simulink model "TeamA_PAsqualo"  (R2020a)
settings: Solver=VariableStepAuto  StartTime=0.0  StopTime=stop_time  FixedStep=0.05  RelTol=1e-3
InitFcn:
  | main_init
values from neighbouring files (symbols this model uses):
  a1 = rho * D^4 * alpha1    (= 0.000388302366464)    [main_init.m]
  a2 = -rho * D^3 * alpha2 * (1 - omega)    (= 0.0037030698432)    [main_init.m]
  ag = [Ax Ay Az]'    [init_modello.m]
  alpha1 = 0.0113    [main_init.m]
  alpha2 = -0.0091    [main_init.m]
  areaOfInterestCorner = [42.317744;10.915136; 0]    [init_controllo.m]    (also in missionA.m = [42.317744)
  bg = [Bx By Bz]'    [init_modello.m]
  cd_pitch = 0.7    [init_modello.m]
  cd_roll = 0.04    [init_modello.m]
  cd_x = 0.4    [init_modello.m]
  cd_y = 1    [init_modello.m]
  cd_yaw = 0.7    [init_modello.m]
  cd_z = 1    [init_modello.m]
  cg = [Cx Cy Cz]'    [init_modello.m]
  D = 0.076    [main_init.m]
  dead_zone_limit = 31.5    [main_init.m]
  dg = [Dx Dy Dz]'    [init_modello.m]
  eg = [Ex Ey Ez]'    [init_modello.m]
  fg = [Fx Fy Fz]'    [init_modello.m]
  g = 9.81    [init_modello.m]
  galleggiamento = 7.6786    [init_controllo.m]
  gg = [Gx Gy Gz]'    [init_modello.m]
  H0 = 0    [init_modello.m]
  init_position = [pointP(1),pointP(2),0.15,0,0,deg2rad(alpha)]'    [init_modello.m]
  init_velocity = [0 0 0 0 0 0]'    [init_modello.m]
  initial_state_cov = blkdiag(diag(cov_gps(1,1:2)), cov_depth*eye(n_state_filter-2))    [init_navigazione.m]
  Ixx = 0.93304097392    [init_modello.m]
  Ixy = 0    [init_modello.m]
  Ixz = 0    [init_modello.m]
  Iyy = 25.58745481378    (= 25.5874548138)    [init_modello.m]
  Iyz = 0    [init_modello.m]
  Izz = 25.58745481378    (= 25.5874548138)    [init_modello.m]
  K_i_heave_div = 20    [init_controllo.m]
  K_i_heave_pos = 1    [init_controllo.m]
  K_i_heave_surf = 20    [init_controllo.m]
  K_i_heave_trans = 5    [init_controllo.m]
  K_i_heave_turn = 5    [init_controllo.m]
  K_i_pitch_div = 0    [init_controllo.m]
  K_i_pitch_pos = 0    [init_controllo.m]
  K_i_pitch_surf = 0    [init_controllo.m]
  K_i_pitch_trans = 0    [init_controllo.m]
  K_i_pitch_turn = 0    [init_controllo.m]
  K_i_roll_div = 0    [init_controllo.m]
  K_i_roll_pos = 0    [init_controllo.m]
  K_i_roll_surf = 1    [init_controllo.m]
  K_i_roll_trans = 0    [init_controllo.m]
  K_i_roll_turn = 0    [init_controllo.m]
  K_i_surge_div = 3    [init_controllo.m]
  K_i_surge_pos = 5    [init_controllo.m]
  K_i_surge_surf = 3    [init_controllo.m]
  K_i_surge_trans = 2.5    [init_controllo.m]
  K_i_surge_turn = 10    [init_controllo.m]
  K_i_sway_div = 6    [init_controllo.m]
  K_i_sway_pos = 5    [init_controllo.m]
  K_i_sway_surf = 3    [init_controllo.m]
  K_i_sway_trans = 6    [init_controllo.m]
  K_i_sway_turn = 50    [init_controllo.m]
  K_i_yaw_div = 0    [init_controllo.m]
  K_i_yaw_pos = 1    [init_controllo.m]
  K_i_yaw_surf = 0    [init_controllo.m]
  K_i_yaw_trans = 20    [init_controllo.m]
  K_p_heave_div = 200    [init_controllo.m]
  K_p_heave_pos = 350    [init_controllo.m]
  K_p_heave_surf = 200    [init_controllo.m]
  K_p_heave_trans = 200    [init_controllo.m]
  K_p_heave_turn = 200    [init_controllo.m]
  K_p_phi_div = 0.15    [init_controllo.m]
  K_p_phi_pos = 0.1    [init_controllo.m]
  K_p_phi_surf = 0.15    [init_controllo.m]
  K_p_phi_trans = 0.1    [init_controllo.m]
  K_p_phi_turn = 0.1    [init_controllo.m]
  K_p_pitch_div = 50    [init_controllo.m]
  K_p_pitch_pos = 25    [init_controllo.m]
  K_p_pitch_surf = 50    [init_controllo.m]
  K_p_pitch_trans = 25    [init_controllo.m]
  K_p_pitch_turn = 25    [init_controllo.m]
  K_p_psi_div = 0.3    [init_controllo.m]
  K_p_psi_pos = 0.25    [init_controllo.m]
  K_p_psi_surf = 0.3    [init_controllo.m]
  K_p_psi_trans = 0.2    [init_controllo.m]
  K_p_roll_div = 10    [init_controllo.m]
  K_p_roll_pos = 4    [init_controllo.m]
  K_p_roll_surf = 10    [init_controllo.m]
  K_p_roll_trans = 4    [init_controllo.m]
  K_p_roll_turn = 4    [init_controllo.m]
  K_p_surge_div = 80    [init_controllo.m]
  K_p_surge_pos = 34.5    [init_controllo.m]
  K_p_surge_surf = 80    [init_controllo.m]
  K_p_surge_trans = 40    [init_controllo.m]
  K_p_surge_turn = 150    [init_controllo.m]
  K_p_sway_div = 100    [init_controllo.m]
  K_p_sway_pos = 90    [init_controllo.m]
  K_p_sway_surf = 80    [init_controllo.m]
  K_p_sway_trans = 90    [init_controllo.m]
  K_p_sway_turn = 200    [init_controllo.m]
  K_p_th_div = 0.3    [init_controllo.m]
  K_p_th_pos = 0.1    [init_controllo.m]
  K_p_th_surf = 0.3    [init_controllo.m]
  K_p_th_trans = 0.1    [init_controllo.m]
  K_p_th_turn = 0.1    [init_controllo.m]
  K_p_x_div = 0.12    [init_controllo.m]
  K_p_x_pos = 0.12    [init_controllo.m]
  K_p_x_surf = 0.12    [init_controllo.m]
  K_p_y_div = 0.6    [init_controllo.m]
  K_p_y_pos = 0.34    [init_controllo.m]
  K_p_y_surf = 0.1    [init_controllo.m]
  K_p_y_trans = 0.3    [init_controllo.m]
  K_p_y_turn = 0.3    [init_controllo.m]
  K_p_yaw_div = 70    [init_controllo.m]
  K_p_yaw_pos = 20    [init_controllo.m]
  K_p_yaw_surf = 70    [init_controllo.m]
  K_p_yaw_trans = 160    [init_controllo.m]
  K_p_z_div = 0.35    [init_controllo.m]
  K_p_z_pos = 0.2    [init_controllo.m]
  K_p_z_surf = 0.35    [init_controllo.m]
  K_p_z_trans = 0.7    [init_controllo.m]
  K_p_z_turn = 0.7    [init_controllo.m]
  Kadd = 0    [init_modello.m]
  m = 106    [init_modello.m]
  Madd = -((((1/5)*(b^2-a^2)^2))*(alpha_0-beta_0))/((((2*(b^2-a^2)^2))+(b^2-a^2)^2)*(alpha_0-beta_0)*m)    [init_modello.m]
  ... (+59 more)
undefined symbols (not defined in the file or in its folder): DiscIntNeverNeededParam, initial_state
libraries: simulink x2, vrlib x1
(part 4 of 5)

== matlab function TeamA_PAsqualo/controller/diving controller/heave_controller/Heave PID controller/compute_position_errors ==
  settings: updateMethod=DISCRETE  sampleTime=0.1
  data: enable input size=1; err_pos output size=1; ref input size=[12 1]; est_state input size=[12 1]; w_des output size=1; areaOfInterestCorner parameter
function [err_pos, w_des] = fcn(enable, ref, est_state,areaOfInterestCorner)
references_NED = zeros(3,1);
est_state_NED  = zeros(3,1);
phi = est_state(4);
th  = est_state(5);
psi = est_state(6);
coder.extrinsic('evalin','wgs84Ellipsoid','geodetic2ned');
orig = [areaOfInterestCorner(1)   areaOfInterestCorner(2)   areaOfInterestCorner(3)]'; %origine terna NED
wgs84 = wgs84Ellipsoid;
err_pos = 0;
w_des = 0;
if enable == 1
    % Cambiamento di riferimento da WGS84 a NED frame
   [x_ref, y_ref, z_ref] = geodetic2ned(ref(1),ref(2),ref(3),orig(1),orig(2),orig(3),wgs84);
   references_NED = [x_ref, y_ref, z_ref]';
   [x_est, y_est, z_est] = geodetic2ned(est_state(1),est_state(2),est_state(3),orig(1),orig(2),orig(3),wgs84);
   est_state_NED  =  [x_est, y_est, z_est]';
   est_state_NED = [est_state_NED(1);est_state_NED(2);est_state(3)];
   % Calcolo errore posizione da NED a BODY frame
   err_NED  = references_NED - est_state_NED;
   R_z_psi = [cos(psi)    sin(psi)     0;
              -sin(psi)   cos(psi)     0;
                 0           0         1];
          
   R_y_th =  [cos(th)        0      -sin(th);
                 0           1         0;
              sin(th)        0       cos(th)];
       
   R_x_phi = [   1           0             0;
                 0         cos(phi)    sin(phi);
                 0        -sin(phi)    cos(phi)];
          
   R_NB = ((R_z_psi')*(R_y_th')*(R_x_phi'))';
   err_pos_BODY = R_NB * err_NED;
   offset = 0.5;  % metri di distanza dal punto desiderato
   if err_pos_BODY(3) > offset
       err_pos = 0;
       w_des   = ref(9);
   end
   if err_pos_BODY(3) <= offset
       err_pos = err_pos_BODY(3);
       w_des   = 0;
   end
else
   err_pos = 0;
   w_des   = 0;
end
end

== stateflow chart TeamA_PAsqualo/Mission Supervisor/Chart ==

== stateflow chart TeamA_PAsqualo/Mission Supervisor/State Management ==
  state Movements [parallel]
    settings: executionOrder=1
    state End [function]
    state positioning
      entry:
      current_state(1:5) = [1 0 0 0 0];
      orBene = 0;
      velNull = 0;
      fromFirstPos = 0;
      during:
      if ~missionEnd %missione appena iniziata
      if ~checkOr([0,0,orDes],orient,errOrPos) && ~orBene
      pos_ref = pointP;
      orient_ref = [0,0,orDes];
      vel_ref = [0,0,0,0,0,0];
      else%orientato bene, dentro o fuori sfera
      orBene=1;
      pos_ref = pointA;
      orient_ref = [0,0,orDes];
      vel_ref = velPos;
      end
      else %missione completata con successo
      pos_ref = pointP;
      orient_ref = [0,0, orDesRit];
      vel_ref = velPos;
      end
    state diving
      entry:
      current_state(1:5) = [0 1 0 0 0];
      velNull = 0;
      during:
      if ~(checkPos(pointA,pos, errSphere) && checkOr([0,0,orDes],orient,errOrPos) ...
      && checkVel(zeros(1,6),[vel(1),vel(2),vel(3),0,0,0],errVelDiv)) && ~velNull
      pos_ref = pointA;
      orient_ref = [0,0,orDes];
      vel_ref = zeros(1,6);
      else
      velNull = 1;
      pos_ref = [pointA(1),pointA(2), pos(3)-(altitude-FLS_down)];
      orient_ref = orientA;
      if (pos_ref(3) - pos(3) > endDiv)
      vel_ref = velSub;
      else
      vel_ref = velRidSub;
      end
      end
    state surfacing
      entry:
      current_state(1:5) = [0 0 0 0 1];
      velNull = 0;
      during:
      if wall || current_state(8)
      pos_ref = [pos(1), pos(2), 0.15];
      else
      if ~checkVel(zeros(1,6),[vel(1),vel(2),vel(3),0,0,0],errVelSurf) && ~velNull
      pos_ref = trWP(nWPTran,:,nTran);
      orient_ref = [0,0,orDesRit];
      vel_ref = zeros(1,6);
      else
      velNull = 1;
      ptSup = trWP(nWPTran,:,nTran);
      pos_ref = [ptSup(1),ptSup(2),0.15];
      orient_ref = [0,0,orDesRit];
      vel_ref = velSurf;
      end
      end
    state transect
      entry:
      current_state(1:5) = [0 0 1 0 0];
      ptx = trWP(wpTR,:,page);
      pos_ref = [ptx(1),ptx(2),pos(3)-(altitude-FLS_down)];
      if mod(page,2) == 0
      orient_ref = orPari;
      else
      orient_ref = orDispari;
      end
      vel_ref = velTran;
      state Disaligned
        (default) -> (junction 490)
        (junction 490) -> (junction 207) : {sizeEmerg = size(wpEmerg);}
        (junction 207) -> (junction 674) [order 1] : [~all(sizeEmerg)]
        (junction 674) -> (junction 681) [order 2] : {wpTR = nWPTran;}
        (junction 207) -> (junction 210) [order 2]
        (junction 674) -> (junction 681) [order 1] : [wpTR + 2 <= nWPTran]
            | {wpTR = wpTR+2;}
        (junction 681) -> (junction 210) : {wpEmerg = currentSwingWaypoints(trWP(wpTR,:,page),pos,distEmerg);}
        (junction 210) -> (junction 396) : {ptx = wpEmerg(idxEmerg,1:3);
            | pos_ref = [ptx(1),ptx(2),pos(3)-(altitude-FLS_down)];
            | vel_ref = vEmergTran;}
        (junction 396) -> (junction 225) [order 1] : [mod(page,2) == 0]
            | {orient_ref = [0 0 angle+180];}
        (junction 396) -> (junction 225) [order 2] : {orient_ref = [0 0 angle];}
        (junction 225) -> (junction 259) [order 2]
        (junction 225) -> (junction 213) [order 1] : [checkPos(pos,pos_ref,errPosWPTrans) &&...
            | checkOr(orient,orient_ref,errOrWPTrans)]
        (junction 213) -> (junction 215) [order 1] : [idxEmerg == length(wpEmerg)]
            | {idxEmerg = 1; current_state(6) = 0;}
        (junction 213) -> (junction 215) [order 2] : {idxEmerg = idxEmerg + 1;}
      state Aligned
        (default) -> (junction 203)
        (junction 203) -> (junction 663) [order 1] : [checkPos(pos_ref,pos,errPosTrans) && checkOr(orient_ref,orient,errOrTrans)]
        (junction 203) -> (junction 219) [order 2]
        (junction 663) -> (junction 219) : [wpTR+1 <= nWPTran]
            | {wpTR = wpTR + 1;} %indica WP successivo
        (junction 219) -> (junction 393) : {wpEmerg =  [];
            | ptx = trWP(wpTR,:,page);
            | pos_ref = [ptx(1),ptx(2),pos(3)-(altitude-FLS_down)];}
        (junction 393) -> (junction 222) [order 1] : [mod(page,2) == 0]
            | {orient_ref = orPari;}
        (junction 393) -> (junction 222) [order 2] : {orient_ref = orDispari;}
        (junction 222) -> (junction 227) [order 1] : [wpTR >= nWPTran - 2]
            | {vel_ref = velRid;}
        (junction 222) -> (junction 227) [order 2] : {vel_ref = velTran;}
      Aligned -> Aligned [order 2]
      Disaligned -> Disaligned [order 2]
      (default) -> Aligned
      Disaligned -> Aligned [order 1] : [~current_state(6)]
      Aligned -> Disaligned [order 1] : [current_state(6)]
    state turn
      entry:
      current_state(1:5) = [0 0 0 1 0];
      state ReferencePoints
        (default) -> (junction 728)
        (junction 728) -> (junction 736) [order 2] : {ptx = turnWP(nWPTurn,:,page);
            | pos_ref = [ptx(1),ptx(2),pos(3)-(altitude-FLS_down)];
            | orient_ref = deg2rad(turnRef(nWPTurn,:,page));}
        (junction 728) -> (junction 733) [order 1] : [time+1<=nWPTurn]
            | {ptx = turnWP(time+1,:,page);
            | pos_ref = [ptx(1),ptx(2),pos(3)-(altitude-FLS_down)];
            | orient_ref = deg2rad(turnRef(time+1,:,page));}
        (junction 736) -> (junction 733)
        (junction 733) -> (junction 738) [order 1] : [mod(page,2) == 0]
            | {vel_ref = [0.2 0 0 0 0 -rot*0.2/(lineSpaceBetweenTransects/2)];}
        (junction 733) -> (junction 731) [order 2] : {vel_ref = [0.2 0 0 0 0 rot*0.2/(lineSpaceBetweenTransects/2)];}
      ReferencePoints -> ReferencePoints
      (default) -> ReferencePoints
    (default) -> positioning : {missionEnd = 0;}
    positioning -> positioning [order 1] : [missionEnd && checkPos(pointP,pos,errPosPos/2)]
        | {End();}
    positioning -> diving [order 2] : [checkPos(pointA,pos,errPosPos) && checkOr([0,0,orDes],orient,errOrPos)]
    positioning -> surfacing [order 3] : [wall || current_state(8)]
        | {fromFirstPos = 1;}
    surfacing -> positioning : [checkPos3([ptSup(1),ptSup(2),0.15],pos,errPosSurf) && ...
        | checkOr([0,0,orDesRit],orient,errOrSurf) && checkVel(zeros(1,6),vel,errVelSurf)...
        | && ~fromFirstPos]
        | {missionEnd = 1;}
    diving -> surfacing [order 2] : [wall || current_state(8)]
    diving -> transect [order 1] : [checkPos3([pointA(1),pointA(2), pos(3)-(altitude-FLS_down)],pos,errPosDiv) ...
        | && checkOr(orientA,orient,errOrDiv)]
    transect -> surfacing [order 1] : [wall || current_state(8)]
    turn -> surfacing [order 2] : [wall || current_state(8)]
    transect -> surfacing [order 2] : [(checkPos(trWP(nWPTran,:,nTran),pos, errPosTrans) &&...
        | checkOr(orient_ref,orient,errOrTrans))]
    turn -> transect [order 1] : [time+1 == nWPTurn]
        | {page = page + 1; wpTR = 1;}
    transect -> turn [order 3] : [checkPos(trWP(nWPTran,:,page),pos, errPosTrans) && checkOr(orient_ref,orient,errOrTrans)]
        | {wpTU=1;}
  state Issues_management [parallel] [commented out]
    entry:
    points=[];
    profs=[];
    state Free [commented out]
      entry:
      current_state(6:8) = 0;
      during:
      if current_state(1) || current_state(5)
      pos_ref(3) = 0.15;
      else
      if abs(altitude - FLS_down)>=0.5
      pos_ref(3)= 30;%pos(3) - (altitude - FLS_down);
      else
      pos_ref(3) = 30;%pos(3);
      end
      end
    state Issue_found [commented out]
      state obstacle %parete/ostacoli [parallel] [commented out]
        during:
        distFront = FLS_front*cos(deg2rad(theta_f));
        distDown = FLS_front*sin(deg2rad(theta_f));
        nedFLS = fix2LocalNED(orient(1),orient(2),orient(3))'*[distFront;0;distDown];
        pointProf = pos(3) - (altitude-FLS_down) - (FLS_down-nedFLS(3));
        pointApp = calcPoint(pos,orient,nedFLS(1));
        nedAxis = (fix2LocalNED(orient(1),orient(2),orient(3))'*[semix; semiy; semiz])';
        if abs(altitude - FLS_down)>=0.5
        pos_ref(3)= pos(3) - (altitude - FLS_down);
        else
        pos_ref(3) = pos(3);
        end
        (default) -> (junction 563) [commented out]
        (junction 563) -> (junction 565) [commented out] : [all(size(points))]
            | {current_state(7) = 1;
            | distObsVeh = distance(pos+nedAxis,points(1,:));}
        (junction 563) -> (junction 575) [commented out] : [~all(size(points))]
            | {current_state(7) = 0;}
        (junction 565) -> (junction 567) [commented out] : [distObsVeh<(abs(pos(3)-profs(1))/maxRatio + safeMargin)]
            | {pos_ref(3) = profs(1);}
        (junction 565) -> (junction 569) [commented out] : [checkRif(pos_ref,orient_ref,vel_ref, ...
            | pos,orient,vel,errPosPos,errOrPos,errVelPos)]
            | {points  = points(2:end,:);}
        (junction 567) -> (junction 573) [commented out]
        (junction 575) -> (junction 573) [commented out]
        (junction 569) -> (junction 573) [commented out]
        (junction 573) -> (junction 578) [commented out] : [(pos(3) - pointProf)/(distFront+nedAxis(1)) > maxRatio]
            | %{current_state(7) = 1;}
            | {wall = 1;}
        (junction 573) -> (junction 605) [commented out]
        (junction 573) -> (junction 580) [commented out] : [(pos(3) - pointProf)/(distFront+nedAxis(1)) <= maxRatio]
        (junction 580) -> (junction 582) [commented out] : [all(size(points))]
            | {distObs = distance(points(end,:),pointApp);}
        (junction 580) -> (junction 586) [commented out] : [pos(3)-pointProf>=minGap]
            | {distObsVeh=distance([pos(1),pos(2)],pointApp)}
        (junction 582) -> (junction 584) [commented out] : [minGap<=abs(profs(end)-pointProf)]
        (junction 586) -> (junction 588) [commented out] : [distObsVeh>=minDist+nedAxis(1)]
            | {points = cat(2,points,pointApp);}
        (junction 584) -> (junction 590) [commented out] : [distObs < minDist || (profs(end)-pointProf)/distObs > maxRatio]
            | {points = points(1:end-1,:);}
        (junction 584) -> (junction 592) [commented out]
        (junction 590) -> (junction 592) [commented out]
        (junction 592) -> (junction 595) [commented out] : {points=cat(1,points,pointApp);}
      state warning %disallineamento [parallel] [commented out]
        during:
        if current_state(3)
        disalignOP;
        end
        if abs(altitude - FLS_down)>=minGap
        pos_ref(3)= pos(3) - (altitude - FLS_down);
        else
        pos_ref(3) = pos(3);
        end
      state abort %danni strutturali [parallel] [commented out]
        entry:
        inactivity = 1;
        during:
        checkFailure;
      state disalignOP [function] [commented out]
        (default) -> (junction 699) [commented out]
        (junction 699) -> (junction 696) [commented out] : {cur_dir = ned2Traj(orient(3))*[1;0;0];
            | err_dir = pos(2) - cur_dir(2);}
        (junction 696) -> (junction 700) [commented out] : [current_state(3) && abs(err_dir)>=offset]
            | {current_state(6) = 1;}
      state checkFailure [function] [commented out]
        (default) -> (junction 108) [commented out]
        (junction 109) -> (junction 114) [commented out] : [mod(inactivity,1000) == 0]
            | {current_state(8) = 1;}
        (junction 108) -> (junction 109) [commented out] : [vel(1:3) == [0 0 0]]
            | {inactivity = inactivity + 1;}
    state rit = check [function] [commented out]
      note: (abs(pos(2)-pos_ref(2))>=offset || abs(pos(1)-pos_ref(1))>=offset))
      (default) -> (junction 690) [commented out]
      (junction 690) -> (junction 122) [commented out] : {cur_dir = ned2Traj(orient(3))*[1;0;0];
          | err_dir = pos(2) - cur_dir(2);}
      (junction 122) -> (junction 479) [commented out] : {rit = 0;}
      (junction 122) -> (junction 124) [commented out] : [(current_state(3) && abs(err_dir)>=offset) || all(size(points)) ]
          | {rit = 1;}%|| checkWall || checkFailure
    (default) -> Free [commented out]
    Free -> Issue_found [commented out] : [check]
    Issue_found -> Free [commented out] : [~check]
  data: puntoDes function_input; puntoCorr function_input; dist function_input; M function_output; vRef function_input; vAct function_input; vErr function_input; okVel function_output; oRef function_input; oAct function_input; oErr function_input; okOr function_output; pRef function_input; pAct function_input; pErr function_input; okPos function_output; pRef function_input; pAct function_input; pErr function_input; okPos function_output; p1 function_input; p2 function_input; valDist function_output; phi function_input; theta function_input; rot function_output; psi function_input; ang function_input; rot function_output; p function_input; o function_input; pt function_output; d function_input; pRef function_input; oRef function_input; vRef function_input; pAct function_input; oAct function_input; vAct function_input; pErr function_input; oErr function_input; vErr function_input; placed function_output; vRef function_input; vAct function_input; vErr function_input; okVel function_output; oRef function_input; oAct function_input; oErr function_input; okOr function_output; pRef function_input; pAct function_input; pErr function_input; okPos function_output; pRef function_input; pAct function_input; pErr function_input; okPos function_output; rit function_output; current_state output size=[1, 8] =[0 0 0 0 0 0 0 0]; pos_ref output =pointP; orient_ref output size=[1 3] =[0 0 deg2rad(angle)]; pos input; orient input; vel input; FLS_front input; FLS_down input; time input; vel_ref output =[0 0 0 0 0 0]; orientA parameter; velPos parameter; velSub parameter; velSurf parameter; velTran parameter; wpEmerg local size=[200 3] =zeros(200,3); altitude parameter; averageDepth parameter; nTran parameter; nWPTran parameter; nWPTurn parameter; pointP parameter; trWP parameter; turnWP parameter; velRid parameter; idxEmerg local =1; missionEnd local =0; endDiv parameter; turnRef parameter; velRidSub parameter; errOrDiv parameter; errOrSurf parameter; errOrTrans parameter; errOrWPTrans parameter; errPosDiv parameter; errPosSurf parameter; errPosTrans parameter; errPosWPTrans parameter; errVelDiv parameter; errVelSurf parameter; inactivity local =1; errOrPos parameter; errPosPos parameter; errVelPos parameter; vEmergTran parameter; angle parameter; offset parameter; sizeEmerg local size=[1,2] =[0 0]; distEmerg parameter; pointA parameter; wpTR local =1; wpTU local =1; page local =1; maxRatio parameter; minDist parameter; minGap parameter; profs local size=[1 20] =zeros(1,20); semix parameter; semiy parameter double; semiz parameter; theta_f parameter; distObsVeh local size=1 =0; distDown local size=1 =0; distFront local size=1 =0; nedAxis local size=[1,3] =zeros(1,3); nedFLS local; pointApp local size=[1,2] =zeros(1,2); pointProf local size=[1 1] =0; points local size=[20 2] =zeros(20,2); distObs local size=1 =0; safeMargin parameter; orDes parameter; orBene local; velNull local; errSphere parameter; ptx local =[0 0 0]; lineSpaceBetweenTransects parameter; ptSup local size=[1 3] =zeros(1,3); orDesRit parameter; orDispari parameter; orPari parameter; fromFirstPos local; wall local =0; cur_dir local; err_dir local; rot parameter
  function M = currentSwingWaypoints(puntoDes,puntoCorr,dist):
    | function  M = currentSwingWaypoints(puntoDes,puntoCorr,dist)
    | %Generazione di waypoint aggiuntivi supponendo di conoscere il punto finale
    | % desiderato sul transetto
    | %
    | %   -puntoDes: punto desiderato sulla traiettoria rettilinea; 1x3 [m m m]
    | %   -puntoCorr: punto stimato di posizione corrente; 1x3 [m m m]
    | %   -dist: distanza tra waypoint; [m]
    | 
    |     %lunghezza segmento
    |     lunghezza= sqrt((puntoCorr(1) - puntoDes(1))^2 +(puntoCorr(2)-puntoDes(2))^2);% + (puntoCorr(3) - puntoDes(3))^2); 
    |     
    |     p = floor(lunghezza/dist); %numero waypoint
    |     
    |     distN = puntoCorr(1) - puntoDes(1); %distanza su N tra punto iniziale e finale
    |     distE = puntoCorr(2) - puntoDes(2); %distanza su E tra punto iniziale e finale
    | %     distD = puntoCorr(3) - puntoDes(3); %distanza su D tra punto iniziale e finale
    |     
    |     deltaE = distE/p; %distanza tra waypoints su East
    |     deltaN = distN/p; %distanza tra waypoints su North
    | %     deltaD = distD/p; %distanza tra waypoints su Down
    |     
    |     matrix = zeros(p-1,3);
    |    
    |     for i = 1:p-1 %possiamo fermarci a p-1 perché waypoint su traiettoria già fornito
    |         waypoint = puntoCorr - i * [deltaN deltaE 0];
    |         waypoint(3) = puntoDes(3);%deltaD];
    |         matrix(i,:) = waypoint;%matrix = cat(1, matrix, waypoint);
    |     end
    |     %matrix = cat(2, matrix, puntoDes);
    |     M = matrix;   
    |    
    | end
  function okVel = checkVel(vRef,vAct,vErr):
    | function okVel = checkVel(vRef,vAct,vErr)
    | %Funzione che controlla che il posizionamento sull'angolo dell'area interessata
    | % sia effettivamente avvenuto, per segnalare l'inizio della fase di
    | % immersione
    | %   -vRef: velocità desiderata; 1x6 [m/s m/s m/s rad/s rad/s rad/s]
    | %   -vAct: velocità corrente; 1x3 [m/s m/s m/s rad/s rad/s rad/s]
    | %   -vErr: errore accettabile in velocità; 1x3 [m/s m/s m/s rad/s rad/s rad/s]
    | 
    |     okVel = all(abs(vRef - vAct) <= vErr); %check su velocità
    | end
  function okOr = checkOr(oRef,oAct,oErr):
    | function okOr = checkOr(oRef,oAct,oErr)
    | %Funzione che controlla che il posizionamento sull'angolo dell'area interessata
    | % sia effettivamente avvenuto, per segnalare l'inizio della fase di
    | % immersione
    | %   -oRef: orientazione desiderata; 1x3 [° ° °]
    | %   -oAct: orientazione corrente, stimata dalla navigazione; 1x3 [° ° °]
    | %   -oErr: errore accettabile in orientamento; 1x3 [° ° °]
    | 
    |     okOr = all(abs(oRef - oAct) <= oErr); %check su orientazione
    | end
  function okPos = checkPos(pRef,pAct,pErr):
    | function okPos = checkPos(pRef,pAct,pErr)
    | %Funzione che controlla che il posizionamento sull'angolo dell'area interessata
    | % sia effettivamente avvenuto, per segnalare l'inizio della fase di
    | % immersione
    | %   -pRef: punto di arrivo desiderato; 1x3 [m m m]
    | %   -pAct: posizione corrente, stimata dalla navigazione; 1x3 [m m m]
    | %   -pErr: errore accettabile in posizione; 1x3 [m m m]
    | 
    |     okPos = all(abs(pRef(1:2) - pAct(1:2))  <= pErr(1:2)); %check su posizione
    | end
  function okPos = checkPos3(pRef,pAct,pErr):
    | function okPos = checkPos3(pRef,pAct,pErr)
    | %Funzione che controlla che il posizionamento sull'angolo dell'area interessata
    | % sia effettivamente avvenuto, per segnalare l'inizio della fase di
    | % immersione
    | %   -pRef: punto di arrivo desiderato; 1x3 [m m m]
    | %   -pAct: posizione corrente, stimata dalla navigazione; 1x3 [m m m]
    | %   -pErr: errore accettabile in posizione; 1x3 [m m m]
    | 
    |     okPos = all(abs(pRef - pAct)  <= pErr); %check su posizione
    | end
  function valDist = distance(p1,p2):
    | function valDist = distance(p1,p2)
    |  %p1,p2 considerati di due dimensioni
    |     valDist = sqrt((p1(1)-p2(1))^2 + (p1(2)-p2(2))^2);
    | end
  function rot = fix2LocalNED(phi, theta, psi):
    | function rot = fix2LocalNED(phi, theta, psi)
    | %Matrice di rotazione generica per una rotazione RPY, da sdr fisso a sdr
    | %ruotato
    | %   -phi: angolo su asse x
    | %   -theta: angolo su asse y
    | %   -psi: angolo su asse z
    | 
    |     phirad = deg2rad(phi);
    |     cr = cos(phirad);
    |     sr = sin(phirad);
    | 
    |     thetarad = deg2rad(theta);
    |     cp = cos(thetarad);
    |     sp = sin(thetarad);
    | 
    |     psirad = deg2rad(psi);
    |     cy = cos(psirad);
    |     sy = sin(psirad);
    | 
    |     rotx = [[1 0 0];
    |             [0 cr sr];
    |             [0 -sr cr]];
    | 
    |     roty = [[cp 0 -sp];
    |             [0 1 0];
    |             [sp 0 cp]];
    | 
    |     rotz = [[cy sy 0];
    |             [-sy cy 0];
    |             [0 0 1]];
    | 
    |     rot = rotx*roty*rotz;
    | 
    | end
  function rot = ned2Traj(ang):
    | function rot = ned2Traj(ang)
    | %Rotation matrix describing the transformation from the local reference
    | %system onto the trajectory to the general NED reference system,
    | %considering a simple yaw rotation
    | %
    | %   -ang: yaw angle; [°]
    | 
    |         a = deg2rad(ang);
    |         rot = [cos(a) sin(a) 0; 
    |                -sin(a) cos(a) 0;
    |                  0 0 1];
    | end
  function pt = calcPoint(p,o,d):
    | function pt = calcPoint(p,o,d)
    |     nedDist = fix2LocalNED(o(1),o(2),o(3))'*[d; 0; 0];
    |     pt = [p(1) p(2)] + [nedDist(1) nedDist(2)];
    |     
    | end
  function placed = checkRif(pRef, oRef, vRef, pAct, oAct, vAct, pErr, oErr, vErr):
    | function placed = checkRif(pRef, oRef, vRef, pAct, oAct, vAct, pErr, oErr, vErr)
    | %Funzione che controlla che il posizionamento sull'angolo dell'area interessata
    | % sia effettivamente avvenuto, per segnalare l'inizio della fase di
    | % immersione
    | %   -pRef: punto di arrivo desiderato; 1x3 [m m m]
    | %   -oRef: orientazione desiderata; 1x3 [° ° °]
    | %   -vRef: velocità desiderata; 1x6 [m/s m/s m/s rad/s rad/s rad/s]
    | %   -pAct: posizione corrente, stimata dalla navigazione; 1x3 [m m m]
    | %   -oAct: orientazione corrente, stimata dalla navigazione; 1x3 [° ° °]
    | %   -vAct: velocità corrente; 1x3 [m/s m/s m/s rad/s rad/s rad/s]
    | %   -pErr: errore accettabile in posizione; 1x3 [m m m]
    | %   -oErr: errore accettabile in orientamento; 1x3 [° ° °]
    | %   -vErr: errore accettabile in velocità; 1x3 [m/s m/s m/s rad/s rad/s rad/s]
    | 
    |     p = abs(pRef - pAct)  <= pErr; %check su posizione
    |     o = abs(oRef - oAct) <= oErr; %check su orientazione
    |     v = abs(vRef - vAct) <= vErr; %check su velocità
    |         
    |     placed = all(p) && all(o) && all(v);
    | 
    | end
  function okVel = checkVel(vRef,vAct,vErr):
    | function okVel = checkVel(vRef,vAct,vErr)
    | %Funzione che controlla che il posizionamento sull'angolo dell'area interessata
    | % sia effettivamente avvenuto, per segnalare l'inizio della fase di
    | % immersione
    | %   -vRef: velocità desiderata; 1x6 [m/s m/s m/s rad/s rad/s rad/s]
    | %   -vAct: velocità corrente; 1x3 [m/s m/s m/s rad/s rad/s rad/s]
    | %   -vErr: errore accettabile in velocità; 1x3 [m/s m/s m/s rad/s rad/s rad/s]
    | 
    |     okVel = all(abs(vRef - vAct) <= vErr); %check su velocità
    | end
  function okOr = checkOr(oRef,oAct,oErr):
    | function okOr = checkOr(oRef,oAct,oErr)
    | %Funzione che controlla che il posizionamento sull'angolo dell'area interessata
    | % sia effettivamente avvenuto, per segnalare l'inizio della fase di
    | % immersione
    | %   -oRef: orientazione desiderata; 1x3 [° ° °]
    | %   -oAct: orientazione corrente, stimata dalla navigazione; 1x3 [° ° °]
    | %   -oErr: errore accettabile in orientamento; 1x3 [° ° °]
    | 
    |     okOr = all(abs(oRef - oAct) <= oErr); %check su orientazione
    | end
  function okPos = checkPos(pRef,pAct,pErr):
    | function okPos = checkPos(pRef,pAct,pErr)
    | %Funzione che controlla che il posizionamento sull'angolo dell'area interessata
    | % sia effettivamente avvenuto, per segnalare l'inizio della fase di
    | % immersione
    | %   -pRef: punto di arrivo desiderato; 1x3 [m m m]
    | %   -pAct: posizione corrente, stimata dalla navigazione; 1x3 [m m m]
    | %   -pErr: errore accettabile in posizione; 1x3 [m m m]
    | 
    |     okPos = all(abs(pRef(1:2) - pAct(1:2))  <= pErr(1:2)); %check su posizione
    | end
  function okPos = checkPos3(pRef,pAct,pErr):
    | function okPos = checkPos3(pRef,pAct,pErr)
    | %Funzione che controlla che il posizionamento sull'angolo dell'area interessata
    | % sia effettivamente avvenuto, per segnalare l'inizio della fase di
    | % immersione
    | %   -pRef: punto di arrivo desiderato; 1x3 [m m m]
    | %   -pAct: posizione corrente, stimata dalla navigazione; 1x3 [m m m]
    | %   -pErr: errore accettabile in posizione; 1x3 [m m m]
    | 
    |     okPos = all(abs(pRef - pAct)  <= pErr); %check su posizione
    | end

== matlab function TeamA_PAsqualo/geo2ned1 ==
  data: geo input; ned output size=[3 1]; ned_origin parameter
function ned = geo2ned(geo, ned_origin)
coder.extrinsic('evalin', 'wgs84Ellipsoid', 'geodetic2ned');

[x, y, ~] = geodetic2ned(geo(1), geo(2), -geo(3),ned_origin(1), ned_origin(2), ned_origin(3), wgs84Ellipsoid);

ned = zeros(3,1);
ned = [x;y;geo(3)];
end

== matlab function TeamA_PAsqualo/Controllo Sbaglia segno su Depth ==
  data: u input size=[3 1]; y output
function y = depth2alt(u)

y = zeros(3,1);

y = u;

y(3) = -u(3);

end

== matlab function TeamA_PAsqualo/Mission Supervisor/Trasf. in NED ==
  data: posArg input; pos output; areaOfInterestCorner parameter
function pos = LLD2NED(posArg,areaOfInterestCorner)
    coder.extrinsic('evalin','wgs84Ellipsoid','geodetic2ned');
    pos = zeros(1,3);
    pos1 = 0;
    pos2 = 0;
    pos3 = 0;
    [pos1, pos2, pos3] = geodetic2ned(posArg(1), posArg(2), posArg(3),areaOfInterestCorner(1), areaOfInterestCorner(2), 0,wgs84Ellipsoid);
    pos = [pos1, pos2, posArg(3)];
end

== matlab function TeamA_PAsqualo/Mission Supervisor/Trasf. in NED1 ==
  data: posArg input; pos output; areaOfInterestCorner parameter
function pos = NED2LLD(posArg,areaOfInterestCorner)
    coder.extrinsic('evalin','wgs84Ellipsoid','ned2geodetic');
    pos = zeros(1,3);
    pos1 = 0;
    pos2 = 0;
    pos3 = 0;
    [pos1, pos2, pos3] = ned2geodetic(posArg(1), posArg(2), posArg(3),areaOfInterestCorner(1), areaOfInterestCorner(2), 0,wgs84Ellipsoid);
    pos = [pos1, pos2, posArg(3)];%-posArg(3)];
end

== matlab function TeamA_PAsqualo/controller/compute n_des ==
  settings: updateMethod=DISCRETE  sampleTime=0.1
  data: enable input size=6; n_des output size=[7 1]; tau_pos input size=6; tau_div input size=6; tau_trans input size=6; tau_turn input size=6; tau_surf input size=6; abort input size=6
function n_des = fcn(enable, tau_pos, tau_div, tau_trans, tau_turn, tau_surf, abort)
j = 0;
tau = zeros(6,1);
for i=1:1:length(enable)
    if enable(i) == 1
        j = i;
    end
end
if j == 1
    tau = tau_pos;
end
if j == 2
    tau = tau_div;
end
if j == 3
    tau = tau_trans;
end
if j == 4
    tau = tau_turn;
end
if j == 5
    tau = tau_surf;
end
if j == 6
    tau = abort;
end
% Definisco la matrice di allocazione ai trust B
p_1 = [0.6  0.15 0.005]';
p_2 = [0.6 -0.15 0.005]';
p_3 = [0  0.2 0]';
p_4 = [0 -0.2 0]';
p_5 = [-1.2  0  0.005]';
p_6 = [-0.9  0  0]';
p_7 = [ 0.9  0  0]';

t_1 = [0 0 1]';
t_2 = [0 0 1]';
t_3 = [1 0 0]';
t_4 = [1 0 0]';
t_5 = [0 0 1]';
t_6 = [0 1 0]';
t_7 = [0 1 0]';

B_1 = [t_1;cross(p_1,t_1)];
B_2 = [t_2;cross(p_2,t_2)];
B_3 = [t_3;cross(p_3,t_3)];
B_4 = [t_4;cross(p_4,t_4)];
B_5 = [t_5;cross(p_5,t_5)];
B_6 = [t_6;cross(p_6,t_6)];
B_7 = [t_7;cross(p_7,t_7)];

B = [B_1 B_2 B_3 B_4 B_5 B_6 B_7];
B_pinv = pinv(B);

% Forze desiderate dei truster

T = B_pinv*tau;

% Conversione delle forze desiderate dei truster in numero di giri
b1 = 0.0003883;
u = T/b1;
offset = 31.5;   %limite della zona morta
n = zeros(7,1);
for i = 1:1:7
    n(i) = sign(u(i))*sqrt(abs(u(i)));
    n(i) = n(i) + sign(n(i))*offset;
end
n_des = n;

== matlab function TeamA_PAsqualo/controller/diving controller/heave_controller/Heave PID controller/compute_velocity_error ==
  settings: updateMethod=DISCRETE  sampleTime=0.1
  data: enable input size=1; err_vel output size=1; v_des input size=1; est_meas input size=[12 1]
function err_vel = fcn(enable,v_des,est_meas)
if enable == 1
   err_vel =  v_des - est_meas(9);
else
    err_vel = 0;
end
end

== matlab function TeamA_PAsqualo/controller/diving controller/pitch_controller/Pitch PID controller/compute_orientation_errors ==
  settings: updateMethod=DISCRETE  sampleTime=0.1
  data: enable input size=1; err_orient output size=1; ref input size=[12 1]; est_state input size=[12 1]
function err_orient = fcn(enable, ref, est_state)
coder.extrinsic('wrapToPi');
err_orient = 0;
phi = est_state(4);
th  = est_state(5);
%
J_inv = [1       0          -sin(th); 
         0   cos(phi)  cos(th)*sin(phi);
         0  -sin(phi)  cos(th)*cos(phi)];
if enable == 1
   err_orient_1 = wrapToPi(J_inv*([ref(4);ref(5);ref(6)] -...
                           [est_state(4);est_state(5);est_state(6)]));
else 
   err_orient_1 = zeros(3,1);
end
err_orient = err_orient_1(2);
end

== matlab function TeamA_PAsqualo/controller/diving controller/pitch_controller/Pitch PID controller/compute_velocity_error ==
  settings: updateMethod=DISCRETE  sampleTime=0.1
  data: enable input size=1; err_vel output size=1; v_des input size=1; est_meas input size=[12 1]
function err_vel = fcn(enable,v_des,est_meas)
if enable == 1
   err_vel =  v_des - est_meas(11);
else
    err_vel = 0;
end
end

== matlab function TeamA_PAsqualo/controller/diving controller/roll_controller/Roll PID controller/compute_orientation_errors ==
  settings: updateMethod=DISCRETE  sampleTime=0.1
  data: enable input size=1; err_orient output size=1; ref input size=[12 1]; est_state input size=[12 1]
function err_orient = fcn(enable, ref, est_state)
coder.extrinsic('wrapToPi');
err_orient = 0;
phi = est_state(4);
th  = est_state(5);
%
J_inv = [1       0          -sin(th); 
         0   cos(phi)  cos(th)*sin(phi);
         0  -sin(phi)  cos(th)*cos(phi)];
if enable == 1
   err_orient_1 = wrapToPi(J_inv*([ref(4);ref(5);ref(6)] -...
                           [est_state(4);est_state(5);est_state(6)]));
else 
   err_orient_1 = zeros(3,1);
end
err_orient = err_orient_1(1);
end

== matlab function TeamA_PAsqualo/controller/diving controller/roll_controller/Roll PID controller/compute_velocity_error ==
  settings: updateMethod=DISCRETE  sampleTime=0.1
  data: enable input size=1; err_vel output size=1; v_des input size=1; est_meas input size=[12 1]
function err_vel = fcn(enable,v_des,est_meas)
if enable == 1
   err_vel =  v_des - est_meas(10);
else
    err_vel = 0;
end
end

== matlab function TeamA_PAsqualo/controller/diving controller/surge_controller/Surge PID controller/compute_position_errors ==
  settings: updateMethod=DISCRETE  sampleTime=0.1
  data: enable input size=1; err_pos output size=1; ref input size=[12 1]; est_state input size=[12 1]; areaOfInterestCorner parameter
function err_pos = fcn(enable, ref, est_state,areaOfInterestCorner)
references_NED = zeros(3,1);
est_state_NED  = zeros(3,1);
phi = est_state(4);
th  = est_state(5);
psi = est_state(6);
coder.extrinsic('evalin','wgs84Ellipsoid','geodetic2ned');
orig = [areaOfInterestCorner(1)   areaOfInterestCorner(2)   areaOfInterestCorner(3)]'; %origine terna NED
wgs84 = wgs84Ellipsoid;
if enable == 1
    % Cambiamento di riferimento da WGS84 a NED frame
   [x_ref, y_ref, z_ref] = geodetic2ned(ref(1),ref(2),ref(3),orig(1),orig(2),orig(3),wgs84);
   references_NED = [x_ref, y_ref, z_ref]';
   [x_est, y_est, z_est] = geodetic2ned(est_state(1),est_state(2),est_state(3),orig(1),orig(2),orig(3),wgs84);
   est_state_NED  =  [x_est, y_est, est_state(3)]';
   % Calcolo errore posizione da NED a BODY frame
   err_NED  = references_NED - est_state_NED;
   R_z_psi = [cos(psi)    sin(psi)     0;
              -sin(psi)   cos(psi)     0;
                 0           0         1];
          
   R_y_th =  [cos(th)        0      -sin(th);
                 0           1         0;
              sin(th)        0       cos(th)];
       
   R_x_phi = [   1           0             0;
                 0         cos(phi)    sin(phi);
                 0        -sin(phi)    cos(phi)];
          
   R_NB = ((R_z_psi')*(R_y_th')*(R_x_phi'))';
   err_pos_BODY = R_NB * err_NED;

   err_pos = err_pos_BODY(1);
else
   err_pos = 0;
end
end

== matlab function TeamA_PAsqualo/controller/diving controller/sway_controller/Sway PID controller/compute_position_errors ==
  settings: updateMethod=DISCRETE  sampleTime=0.1
  data: enable input size=1; err_pos output size=1; ref input size=[12 1]; est_state input size=[12 1]; areaOfInterestCorner parameter
function err_pos = fcn(enable, ref, est_state,areaOfInterestCorner)
references_NED = zeros(3,1);
est_state_NED  = zeros(3,1);
phi = est_state(4);
th  = est_state(5);
psi = est_state(6);
coder.extrinsic('evalin','wgs84Ellipsoid','geodetic2ned');
orig = [areaOfInterestCorner(1)   areaOfInterestCorner(2)   areaOfInterestCorner(3)]'; %origine terna NED
wgs84 = wgs84Ellipsoid;
if enable == 1
    % Cambiamento di riferimento da WGS84 a NED frame
   [x_ref, y_ref, z_ref] = geodetic2ned(ref(1),ref(2),ref(3),orig(1),orig(2),orig(3),wgs84);
   references_NED = [x_ref, y_ref, z_ref]';
   [x_est, y_est, z_est] = geodetic2ned(est_state(1),est_state(2),est_state(3),orig(1),orig(2),orig(3),wgs84);
   est_state_NED  = [x_est, y_est, est_state(3)]';
   % Calcolo errore posizione da NED a BODY frame
   err_NED  = references_NED - est_state_NED;
   R_z_psi = [cos(psi)    sin(psi)     0;
              -sin(psi)   cos(psi)     0;
                 0           0         1];
          
   R_y_th =  [cos(th)        0      -sin(th);
                 0           1         0;
              sin(th)        0       cos(th)];
       
   R_x_phi = [   1           0             0;
                 0         cos(phi)    sin(phi);
                 0        -sin(phi)    cos(phi)];
          
   R_NB = ((R_z_psi')*(R_y_th')*(R_x_phi'))';
   err_pos_BODY = R_NB * err_NED;
   err_pos = err_pos_BODY(2);
else
   err_pos = 0;
end
end

== matlab function TeamA_PAsqualo/controller/diving controller/sway_controller/Sway PID controller/compute_velocity_error ==
  settings: updateMethod=DISCRETE  sampleTime=0.1
  data: enable input size=1; err_vel output size=1; v_des input size=1; est_meas input size=[12 1]
function err_vel = fcn(enable,v_des,est_meas)
if enable == 1
   err_vel =  v_des - est_meas(8);
else
    err_vel = 0;
end
end

== matlab function TeamA_PAsqualo/controller/diving controller/yaw_controller/Yaw PID controller/compute_orientation_errors ==
  settings: updateMethod=DISCRETE  sampleTime=0.1
  data: enable input size=1; err_orient output size=1; ref input size=[12 1]; est_state input size=[12 1]
function err_orient = fcn(enable, ref, est_state)
coder.extrinsic('wrapToPi');
err_orient = 0;
phi = est_state(4);
th  = est_state(5);
%
J_inv = [1       0          -sin(th); 
         0   cos(phi)  cos(th)*sin(phi);
         0  -sin(phi)  cos(th)*cos(phi)];
if enable == 1
   err_orient_1 = wrapToPi(J_inv*([ref(4);ref(5);ref(6)] -...
                           [est_state(4);est_state(5);est_state(6)]));
else 
   err_orient_1 = zeros(3,1);
end
err_orient = err_orient_1(3);
end

== matlab function TeamA_PAsqualo/controller/diving controller/surge_controller/Surge PID controller/compute_velocity_error ==
  settings: updateMethod=DISCRETE  sampleTime=0.1
  data: enable input size=1; err_vel output size=1; v_des input size=1; est_meas input size=[12 1]
function err_vel = fcn(enable,v_des,est_meas)
if enable == 1
   err_vel =  v_des - est_meas(7);
else
    err_vel = 0;
end
end

== matlab function TeamA_PAsqualo/controller/diving controller/yaw_controller/Yaw PID controller/compute_velocity_error ==
  data: enable input; err_vel output; v_des input; est_meas input
function err_vel = fcn(enable,v_des,est_meas)
if enable == 1
   err_vel =  v_des - est_meas(12);
else
    err_vel = 0;
end

== matlab function TeamA_PAsqualo/controller/positioning controller/heave_controller/Heave PID controller/compute_position_errors ==
  data: enable input; err_pos output; ref input; est_state input; areaOfInterestCorner parameter
function err_pos = fcn(enable, ref, est_state,areaOfInterestCorner)
references_NED = zeros(3,1);
est_state_NED  = zeros(3,1);
phi = est_state(4);
th  = est_state(5);
psi = est_state(6);
coder.extrinsic('evalin','wgs84Ellipsoid','geodetic2ned');   
orig = [areaOfInterestCorner(1)   areaOfInterestCorner(2)   areaOfInterestCorner(3)]'; %origine terna NED
wgs84 = wgs84Ellipsoid;
if enable == 1
    % Cambiamento di riferimento da WGS84 a NED frame
   [x_ref, y_ref, z_ref] = geodetic2ned(ref(1),ref(2),ref(3),orig(1),orig(2),orig(3),wgs84);
   references_NED = [x_ref, y_ref, z_ref]';
   [x_est, y_est, z_est] = geodetic2ned(est_state(1),est_state(2),est_state(3),orig(1),orig(2),orig(3),wgs84);
   est_state_NED  =  [x_est, y_est, est_state(3)]';
   % Calcolo errore posizione da NED a BODY frame
   err_NED  = references_NED - est_state_NED;
   R_z_psi = [cos(psi)    sin(psi)     0;
              -sin(psi)   cos(psi)     0;
                 0           0         1];
          
   R_y_th =  [cos(th)        0      -sin(th);
                 0           1         0;
              sin(th)        0       cos(th)];
       
   R_x_phi = [   1           0             0;
                 0         cos(phi)    sin(phi);
                 0        -sin(phi)    cos(phi)];
          
   R_NB = ((R_z_psi')*(R_y_th')*(R_x_phi'))';
   err_pos_BODY = R_NB * err_NED;
   err_pos = err_pos_BODY(3);
else
   err_pos = 0;
end
end

== matlab function TeamA_PAsqualo/controller/positioning controller/heave_controller/Heave PID controller/compute_velocity_error ==
  data: enable input; err_vel output; v_des input; est_meas input
function err_vel = fcn(enable,v_des,est_meas)
err_vel = 0;
if enable == 1
   err_vel =  v_des - est_meas(9);
else 
    err_vel = 0;
end
end

== matlab function TeamA_PAsqualo/controller/positioning controller/pitch_controller/Pitch PID controller/compute_orientation_errors ==
  data: enable input; err_orient output; ref input; est_state input
function err_orient = fcn(enable, ref, est_state)
coder.extrinsic('wrapToPi');
err_orient = 0;
phi = est_state(4);
th  = est_state(5);
%
J_inv = [1       0          -sin(th); 
         0   cos(phi)  cos(th)*sin(phi);
         0  -sin(phi)  cos(th)*cos(phi)];
if enable == 1
   err_orient_1 = wrapToPi(J_inv*([ref(4);ref(5);ref(6)] -...
                                [est_state(4);est_state(5);est_state(6)]));
else 
   err_orient_1 = zeros(3,1);
end
err_orient = err_orient_1(2);
end

== matlab function TeamA_PAsqualo/controller/positioning controller/pitch_controller/Pitch PID controller/compute_velocity_error ==
  data: enable input; err_vel output; v_des input; est_meas input
function err_vel = fcn(enable,v_des,est_meas)
if enable == 1
   err_vel =  v_des - est_meas(11);
else
    err_vel = 0;
end
end

== matlab function TeamA_PAsqualo/controller/positioning controller/roll_controller/Roll PID controller/compute_orientation_errors ==
  data: enable input; err_orient output; ref input; est_state input
function err_orient = fcn(enable, ref, est_state)
coder.extrinsic('wrapToPi');
err_orient = 0;
phi = est_state(4);
th  = est_state(5);
%
J_inv = [1       0          -sin(th); 
         0   cos(phi)  cos(th)*sin(phi);
         0  -sin(phi)  cos(th)*cos(phi)];
if enable == 1
   err_orient_1 = wrapToPi(J_inv*([ref(4);ref(5);ref(6)] -...
                           [est_state(4);est_state(5);est_state(6)]));
else 
   err_orient_1 = zeros(3,1);
end
err_orient = err_orient_1(1);
end

== matlab function TeamA_PAsqualo/controller/positioning controller/roll_controller/Roll PID controller/compute_velocity_error ==
  data: enable input; err_vel output; v_des input; est_meas input
function err_vel = fcn(enable,v_des,est_meas)
if enable == 1
   err_vel =  v_des - est_meas(10);
else 
    err_vel = 0;
end
end

== matlab function TeamA_PAsqualo/controller/positioning controller/surge_controller/Surge PID controller/compute_position_errors ==
  data: enable input; err_pos output; ref input; est_state input; u_des output; areaOfInterestCorner parameter
function [err_pos, u_des] = fcn(enable, ref, est_state,areaOfInterestCorner)
references_NED = zeros(3,1);
est_state_NED  = zeros(3,1);
phi = est_state(4);
th  = est_state(5);
psi = est_state(6);
coder.extrinsic('evalin','wgs84Ellipsoid','geodetic2ned');
orig = [areaOfInterestCorner(1)   areaOfInterestCorner(2)   areaOfInterestCorner(3)]'; %origine terna NED
wgs84 = wgs84Ellipsoid;
err_pos = 0;
u_des = 0;

if enable == 1
    % Cambiamento di riferimento da WGS84 a NED frame
   [x_ref, y_ref, z_ref] = geodetic2ned(ref(1),ref(2),ref(3),orig(1),orig(2),orig(3),wgs84);
   references_NED = [x_ref, y_ref, z_ref]';
   [x_est, y_est, z_est] = geodetic2ned(est_state(1),est_state(2),est_state(3),orig(1),orig(2),orig(3),wgs84);
   est_state_NED  =  [x_est, y_est, z_est]';
   est_state_NED = [est_state_NED(1);est_state_NED(2);est_state(3)];
   % Calcolo errore posizione da NED a BODY frame
   err_NED  = references_NED - est_state_NED;
   R_z_psi = [cos(psi)    sin(psi)     0;
              -sin(psi)   cos(psi)     0;
                 0           0         1];
          
   R_y_th =  [cos(th)        0      -sin(th);
                 0           1         0;
              sin(th)        0       cos(th)];
       
   R_x_phi = [   1           0             0;
                 0         cos(phi)    sin(phi);
                 0        -sin(phi)    cos(phi)];
          
   R_NB = ((R_z_psi')*(R_y_th')*(R_x_phi'))';
   err_pos_BODY = R_NB * err_NED;
   offset = 5;  % metri di distanza dal punto desiderato
   if abs(err_pos_BODY(1)) > offset
       err_pos = 0;
       u_des   = ref(7);
   end
   if abs(err_pos_BODY(1)) <= offset
       err_pos = err_pos_BODY(1);
       u_des   = 0;
   end
else
   err_pos = 0;
   u_des   = 0;
end
end

== matlab function TeamA_PAsqualo/controller/positioning controller/surge_controller/Surge PID controller/compute_velocity_error ==
  data: enable input; err_vel output; v_des input; est_meas input
function err_vel = fcn(enable,v_des,est_meas)
if enable == 1
   err_vel =  v_des - est_meas(7);
else
    err_vel = 0;
end
end
